simulink model "PassStFtIsPosChk"  (R2024b)
settings: Solver=FixedStepDiscrete  StartTime=0.0  StopTime=10.0  FixedStep=0.01  RelTol=1e-3
model workspace (MAT data in the model file):
  KeSMSuFirstRwStBackPosDelta_Val = Simulink.Parameter
  KeSMSuFirstRwStBackPosDelta_Val.Value = 150
  KeSMSuFirstRwStBackPosDelta_Val.Complexity = 'real'
  KeSMSuFirstRwStBackPosDelta_Val.Dimensions = [1 1]
  KeSMSuFirstRwStBackPosDelta_Val.DataType = 'uint16'
  KeSMSuFirstRwStBackPosTolr_Val = Simulink.Parameter
  KeSMSuFirstRwStBackPosTolr_Val.Value = 150
  KeSMSuFirstRwStBackPosTolr_Val.Complexity = 'real'
  KeSMSuFirstRwStBackPosTolr_Val.Dimensions = [1 1]
  KeSMSuFirstRwStBackPosTolr_Val.DataType = 'uint16'
  KeSMSwAcsMd1PassStCshnRrUpwdDnwdPosMax_Val = Simulink.Parameter
  KeSMSwAcsMd1PassStCshnRrUpwdDnwdPosMax_Val.Value = 0
  KeSMSwAcsMd1PassStCshnRrUpwdDnwdPosMax_Val.Complexity = 'real'
  KeSMSwAcsMd1PassStCshnRrUpwdDnwdPosMax_Val.Dimensions = [1 1]
  KeSMSwAcsMd1PassStCshnRrUpwdDnwdPosMax_Val.DataType = 'uint16'
  KeSMSwAcsMd1PassStCshnRrUpwdDnwdPosMin_Val = Simulink.Parameter
  KeSMSwAcsMd1PassStCshnRrUpwdDnwdPosMin_Val.Value = 0
  KeSMSwAcsMd1PassStCshnRrUpwdDnwdPosMin_Val.Complexity = 'real'
  KeSMSwAcsMd1PassStCshnRrUpwdDnwdPosMin_Val.Dimensions = [1 1]
  KeSMSwAcsMd1PassStCshnRrUpwdDnwdPosMin_Val.DataType = 'uint16'
  KeSMSwAcsMd1PassStCshnRrUpwdDnwdPos_Val = Simulink.Parameter
  KeSMSwAcsMd1PassStCshnRrUpwdDnwdPos_Val.Value = 0
  KeSMSwAcsMd1PassStCshnRrUpwdDnwdPos_Val.Complexity = 'real'
  KeSMSwAcsMd1PassStCshnRrUpwdDnwdPos_Val.Dimensions = [1 1]
  KeSMSwAcsMd1PassStCshnRrUpwdDnwdPos_Val.DataType = 'uint16'
  KeSMSwAcsMd56PassStCshnRrUpwdDnwdPosMax_Val = Simulink.Parameter
  KeSMSwAcsMd56PassStCshnRrUpwdDnwdPosMax_Val.Value = 0
  KeSMSwAcsMd56PassStCshnRrUpwdDnwdPosMax_Val.Complexity = 'real'
  KeSMSwAcsMd56PassStCshnRrUpwdDnwdPosMax_Val.Dimensions = [1 1]
  KeSMSwAcsMd56PassStCshnRrUpwdDnwdPosMax_Val.DataType = 'uint16'
  KeSMSwAcsMd56PassStCshnRrUpwdDnwdPosMin_Val = Simulink.Parameter
  KeSMSwAcsMd56PassStCshnRrUpwdDnwdPosMin_Val.Value = 0
  KeSMSwAcsMd56PassStCshnRrUpwdDnwdPosMin_Val.Complexity = 'real'
  KeSMSwAcsMd56PassStCshnRrUpwdDnwdPosMin_Val.Dimensions = [1 1]
  KeSMSwAcsMd56PassStCshnRrUpwdDnwdPosMin_Val.DataType = 'uint16'
  KeSMSwAcsMd56PassStCshnRrUpwdDnwdPos_Val = Simulink.Parameter
  KeSMSwAcsMd56PassStCshnRrUpwdDnwdPos_Val.Value = 0
  KeSMSwAcsMd56PassStCshnRrUpwdDnwdPos_Val.Complexity = 'real'
  KeSMSwAcsMd56PassStCshnRrUpwdDnwdPos_Val.Dimensions = [1 1]
  KeSMSwAcsMd56PassStCshnRrUpwdDnwdPos_Val.DataType = 'uint16'
undefined symbols (not defined in the file or in its folder): KeSMSuFirstRwStFootrestPosDelta_Val, KeSMSuFirstRwStFootrestPosTolr_Val
libraries: simulink x5, StIsPosChkLib x4
settings Model: ParameterArgumentNames=KeSMSuFirstRwStBackPosDelta_Val,KeSMSuFirstRwStBackPosTolr_Val,KeSMSwAcsMd1PassStCshnRrUpwdDnwdPosMax_Val,KeSMSwAcsMd1PassStCshnRrUpwdDnwdPosMin_Val,KeSMSwAcsMd1PassStCshnRrUpwdDnwdPos_Val,KeSMSwAcsMd56PassStCshnRrUpwdDnwdPosMax_Val,KeSMSwAcsMd56PassStCshnRrUpwdDnwdPosMin_Val,KeSMSwAcsMd56PassStCshnRrUpwdDnwdPos_Val  Creator=sn2xws  LastModifiedBy=sn55gm
settings SolverCC: AlgebraicLoopSolver=TrustRegion
settings DataIOCC: SaveFormat=StructureWithTime  ReturnWorkspaceOutputs=off
settings OptimizationCC: DefaultParameterBehavior=Inlined  EnhancedBackFolding=on  PassReuseOutputArgsAs=Individual arguments  ZeroExternalMemoryAtStartup=off  ZeroInternalMemoryAtStartup=off  OptimizeBlockOrder=speed  DifferentSizesBufferReuse=on  OptimizationCustomize=off  EfficientTunableParamExpr=on
settings DebuggingCC: ParameterTunabilityLossMsg=error  UnconnectedInputMsg=warning  UnconnectedOutputMsg=warning  UnconnectedLineMsg=warning  ArithmeticOperatorsInVariantConditions=warning
settings ModelReferenceCC: EnableRefExpFcnMdlSchedulingChecks=on  ModelReferenceNumInstancesAllowed=Single
settings SFSimCC: MATLABDynamicMemAlloc=off  CustomCodeUndefinedFunction=UseInterfaceOnly
settings RTWCC: Description=AUTOSAR  SystemTargetFile=autosar.tlc  GenCodeOnly=on  TemplateMakefile=ert_default_tmf  GenerateReport=on  IncludeHyperlinkInReport=on  LaunchReport=on  DataTypeReplacement=CDataTypesFixedWidth  GenerateTraceInfo=on  GenerateTraceReport=on  GenerateTraceReportSl=on  GenerateTraceReportSf=on  GenerateTraceReportEml=on  GenerateCodeMetricsReport=on  GPUComputeCapability=3.5
settings CodeAppCC: ForceParamTrailComments=on  IgnoreCustomStorageClasses=off  OperatorAnnotations=on  SimulinkDataObjDesc=on  SFDataObjDesc=on  InsertBlockDesc=on
settings STFCustomTargetCC: TargetLangStandard=C99 (ISO)  MultiwordLength=256  ParMdlRefBuildCompliant=on  CompOptLevelCompliant=on  IncludeMdlTerminateFcn=off  CombineOutputUpdateFcns=on  SuppressErrorStatus=on  ERTCustomFileBanners=on  SupportNonFinite=off  SupportComplex=off  SupportContinuousTime=off  SupportNonInlinedSFcns=off  RemoveResetFunc=on  MATLABClassNameForMDSCustomization=Simulink.SoftwareTarget.ERTCustomization  AutosarCompliant=on  UseToolchainInfoCompliant=on  LookupTableObjectStructAxisOrder=2,1,3,4,...  LUTObjectStructOrderEvenSpacing=Size,Table,Breakpoints  SystemTargetFile=autosar.tlc
settings ERTTargetCC: TargetLangStandard=C99 (ISO)  ConcurrentExecutionCompliant=off  IncludeMdlTerminateFcn=off  SuppressErrorStatus=on  SupportNonFinite=off  SupportComplex=off  ModelStepFunctionPrototypeControlCompliant=off  CPPClassGenCompliant=off  AutosarCompliant=on  LookupTableObjectStructAxisOrder=2,1,3,4,...  LUTObjectStructOrderEvenSpacing=Size,Table,Breakpoints  ERTCustomFileTemplate=example_file_process.tlc  ERTFilePackagingFormat=Compact  BooleanTrueId=TRUE  BooleanFalseId=FALSE  DynamicArrayContainerType=coder::array

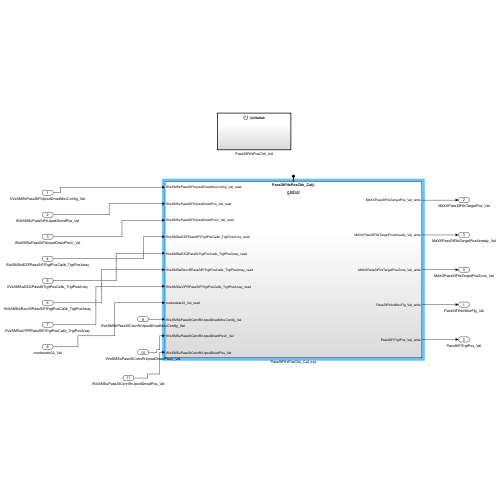
[thumbnail: Simulink's stored preview of the top-level diagram]
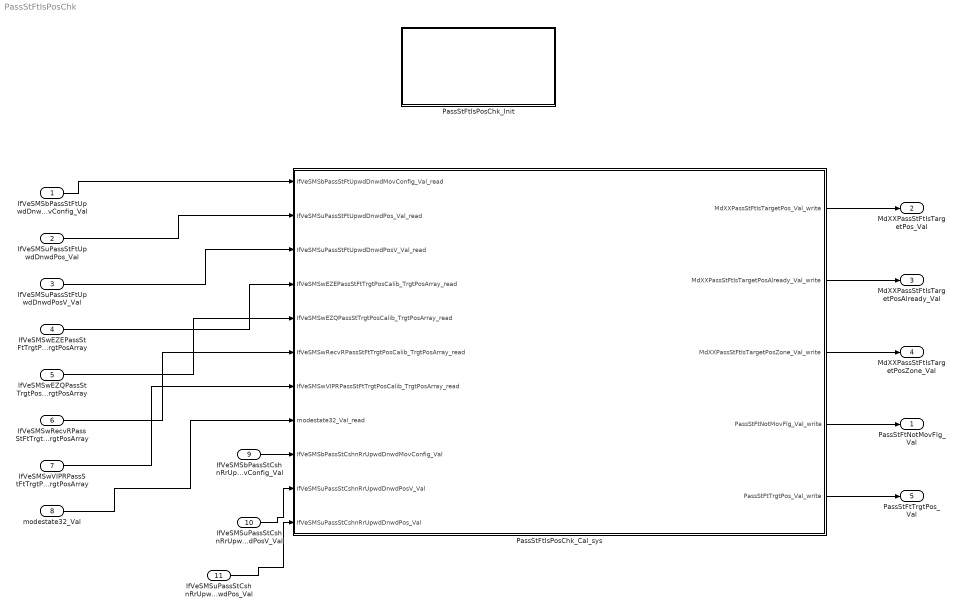
== system PassStFtIsPosChk ==
  IfVeSMSbPassStFtUpwdDnwdMovConfig_Val : Inport  OutDataTypeStr=boolean  PortDimensions=1
  IfVeSMSuPassStFtUpwdDnwdPos_Val : Inport  Port=2  OutDataTypeStr=uint16  PortDimensions=1
  IfVeSMSuPassStFtUpwdDnwdPosV_Val : Inport  Port=3  OutDataTypeStr=boolean  PortDimensions=1
  IfVeSMSwEZEPassStFtTrgtPosCalib_TrgtPosArray : Inport  Description=|  Port=4  OutDataTypeStr=uint16  PortDimensions=3
      | 0:Pos
      | 1:Max
      | 2:Min
  IfVeSMSwEZQPassStTrgtPosCalib_TrgtPosArray : Inport  Description=|  Port=5  OutDataTypeStr=uint16  PortDimensions=3
      | 0:Pos
      | 1:Max
      | 2:Min
  IfVeSMSwRecvRPassStFtTrgtPosCalib_TrgtPosArray : Inport  Description=|  Port=6  OutDataTypeStr=uint16  PortDimensions=3
      | 0:Pos
      | 1:Max
      | 2:Min
  IfVeSMSwVIPRPassStFtTrgtPosCalib_TrgtPosArray : Inport  Description=|  Port=7  OutDataTypeStr=uint16  PortDimensions=3
      | 0:Pos
      | 1:Max
      | 2:Min
  modestate32_Val : Inport  Port=8  OutDataTypeStr=uint32  PortDimensions=1
  IfVeSMSbPassStCshnRrUpwdDnwdMovConfig_Val : Inport  Port=9  OutDataTypeStr=boolean  PortDimensions=1
  IfVeSMSuPassStCshnRrUpwdDnwdPosV_Val : Inport  Port=10  OutDataTypeStr=boolean  PortDimensions=1
  IfVeSMSuPassStCshnRrUpwdDnwdPos_Val : Inport  Port=11  OutDataTypeStr=uint16  PortDimensions=1
  PassStFtIsPosChk_Cal_sys : Subsystem
  PassStFtIsPosChk_Init : Subsystem
  PassStFtNotMovFlg_Val : Outport  OutDataTypeStr=boolean  PortDimensions=1  VectorParamsAs1DForOutWhenUnconnected=off
  MdXXPassStFtIsTargetPos_Val : Outport  Port=2  OutDataTypeStr=uint32  PortDimensions=1  VectorParamsAs1DForOutWhenUnconnected=off
  MdXXPassStFtIsTargetPosAlready_Val : Outport  Port=3  OutDataTypeStr=uint32  PortDimensions=1  VectorParamsAs1DForOutWhenUnconnected=off
  MdXXPassStFtIsTargetPosZone_Val : Outport  Port=4  OutDataTypeStr=uint32  PortDimensions=1  VectorParamsAs1DForOutWhenUnconnected=off
  PassStFtTrgtPos_Val : Outport  Port=5  OutDataTypeStr=uint16  PortDimensions=1  VectorParamsAs1DForOutWhenUnconnected=off
  wires:
  PassStFtIsPosChk_Cal_sys/3(MdXXPassStFtIsTargetPosZone_Val_write) -> MdXXPassStFtIsTargetPosZone_Val/1
  PassStFtIsPosChk_Cal_sys/5(PassStFtTrgtPos_Val_write) -> PassStFtTrgtPos_Val/1
  IfVeSMSuPassStFtUpwdDnwdPosV_Val/1 -> PassStFtIsPosChk_Cal_sys/3(IfVeSMSuPassStFtUpwdDnwdPosV_Val_read)
  IfVeSMSuPassStFtUpwdDnwdPos_Val/1 -> PassStFtIsPosChk_Cal_sys/2(IfVeSMSuPassStFtUpwdDnwdPos_Val_read)
  IfVeSMSwEZEPassStFtTrgtPosCalib_TrgtPosArray/1 -> PassStFtIsPosChk_Cal_sys/4(IfVeSMSwEZEPassStFtTrgtPosCalib_TrgtPosArray_read)
  IfVeSMSbPassStFtUpwdDnwdMovConfig_Val/1 -> PassStFtIsPosChk_Cal_sys/1(IfVeSMSbPassStFtUpwdDnwdMovConfig_Val_read)
  IfVeSMSwEZQPassStTrgtPosCalib_TrgtPosArray/1 -> PassStFtIsPosChk_Cal_sys/5(IfVeSMSwEZQPassStTrgtPosCalib_TrgtPosArray_read)
  IfVeSMSwRecvRPassStFtTrgtPosCalib_TrgtPosArray/1 -> PassStFtIsPosChk_Cal_sys/6(IfVeSMSwRecvRPassStFtTrgtPosCalib_TrgtPosArray_read)
  IfVeSMSwVIPRPassStFtTrgtPosCalib_TrgtPosArray/1 -> PassStFtIsPosChk_Cal_sys/7(IfVeSMSwVIPRPassStFtTrgtPosCalib_TrgtPosArray_read)
  modestate32_Val/1 -> PassStFtIsPosChk_Cal_sys/8(modestate32_Val_read)
  PassStFtIsPosChk_Cal_sys/1(MdXXPassStFtIsTargetPos_Val_write) -> MdXXPassStFtIsTargetPos_Val/1
  PassStFtIsPosChk_Cal_sys/2(MdXXPassStFtIsTargetPosAlready_Val_write) -> MdXXPassStFtIsTargetPosAlready_Val/1
  PassStFtIsPosChk_Cal_sys/4(PassStFtNotMovFlg_Val_write) -> PassStFtNotMovFlg_Val/1
  IfVeSMSbPassStCshnRrUpwdDnwdMovConfig_Val/1 -> PassStFtIsPosChk_Cal_sys/9(IfVeSMSbPassStCshnRrUpwdDnwdMovConfig_Val)
  IfVeSMSuPassStCshnRrUpwdDnwdPosV_Val/1 -> PassStFtIsPosChk_Cal_sys/10(IfVeSMSuPassStCshnRrUpwdDnwdPosV_Val)
  IfVeSMSuPassStCshnRrUpwdDnwdPos_Val/1 -> PassStFtIsPosChk_Cal_sys/11(IfVeSMSuPassStCshnRrUpwdDnwdPos_Val)

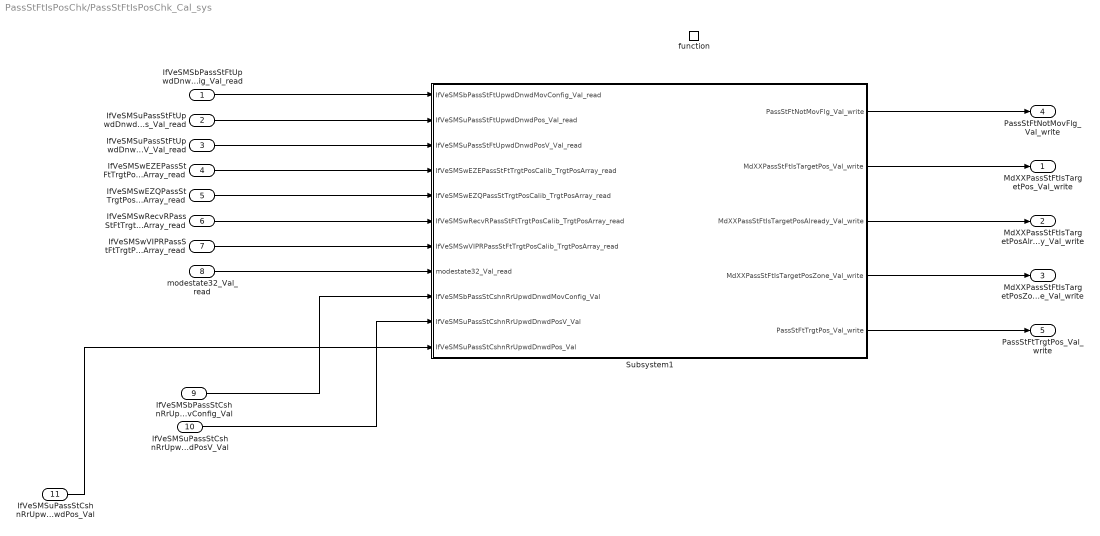
== system PassStFtIsPosChk/PassStFtIsPosChk_Cal_sys ==
  IfVeSMSbPassStFtUpwdDnwdMovConfig_Val_read : Inport
  IfVeSMSuPassStFtUpwdDnwdPos_Val_read : Inport  Port=2
  IfVeSMSuPassStFtUpwdDnwdPosV_Val_read : Inport  Port=3
  IfVeSMSwEZEPassStFtTrgtPosCalib_TrgtPosArray_read : Inport  Port=4
  IfVeSMSwEZQPassStTrgtPosCalib_TrgtPosArray_read : Inport  Port=5
  IfVeSMSwRecvRPassStFtTrgtPosCalib_TrgtPosArray_read : Inport  Port=6
  IfVeSMSwVIPRPassStFtTrgtPosCalib_TrgtPosArray_read : Inport  Port=7
  modestate32_Val_read : Inport  Port=8
  IfVeSMSbPassStCshnRrUpwdDnwdMovConfig_Val : Inport  Port=9
  IfVeSMSuPassStCshnRrUpwdDnwdPosV_Val : Inport  Port=10
  IfVeSMSuPassStCshnRrUpwdDnwdPos_Val : Inport  Port=11
  function : TriggerPort  TriggerType=function-call  IsSimulinkFunction=on  FunctionName=PassStFtIsPosChk_Cal  VariantControl=(inherit)
  Subsystem1 : Subsystem
  MdXXPassStFtIsTargetPos_Val_write : Outport  VectorParamsAs1DForOutWhenUnconnected=off
      settings: EnsureOutportIsVirtual=on
  MdXXPassStFtIsTargetPosAlready_Val_write : Outport  Port=2  VectorParamsAs1DForOutWhenUnconnected=off
      settings: EnsureOutportIsVirtual=on
  MdXXPassStFtIsTargetPosZone_Val_write : Outport  Port=3  VectorParamsAs1DForOutWhenUnconnected=off
      settings: EnsureOutportIsVirtual=on
  PassStFtNotMovFlg_Val_write : Outport  Port=4  VectorParamsAs1DForOutWhenUnconnected=off
      settings: EnsureOutportIsVirtual=on
  PassStFtTrgtPos_Val_write : Outport  Port=5  VectorParamsAs1DForOutWhenUnconnected=off
      settings: EnsureOutportIsVirtual=on
  wires:
  IfVeSMSwEZQPassStTrgtPosCalib_TrgtPosArray_read/1 -> Subsystem1/5(IfVeSMSwEZQPassStTrgtPosCalib_TrgtPosArray_read)
  IfVeSMSwRecvRPassStFtTrgtPosCalib_TrgtPosArray_read/1 -> Subsystem1/6(IfVeSMSwRecvRPassStFtTrgtPosCalib_TrgtPosArray_read)
  IfVeSMSuPassStFtUpwdDnwdPosV_Val_read/1 -> Subsystem1/3(IfVeSMSuPassStFtUpwdDnwdPosV_Val_read)
  IfVeSMSwEZEPassStFtTrgtPosCalib_TrgtPosArray_read/1 -> Subsystem1/4(IfVeSMSwEZEPassStFtTrgtPosCalib_TrgtPosArray_read)
  IfVeSMSwVIPRPassStFtTrgtPosCalib_TrgtPosArray_read/1 -> Subsystem1/7(IfVeSMSwVIPRPassStFtTrgtPosCalib_TrgtPosArray_read)
  IfVeSMSuPassStFtUpwdDnwdPos_Val_read/1 -> Subsystem1/2(IfVeSMSuPassStFtUpwdDnwdPos_Val_read)
  modestate32_Val_read/1 -> Subsystem1/8(modestate32_Val_read)
  IfVeSMSbPassStFtUpwdDnwdMovConfig_Val_read/1 -> Subsystem1/1(IfVeSMSbPassStFtUpwdDnwdMovConfig_Val_read)
  Subsystem1/1(PassStFtNotMovFlg_Val_write) -> PassStFtNotMovFlg_Val_write/1
  Subsystem1/2(MdXXPassStFtIsTargetPos_Val_write) -> MdXXPassStFtIsTargetPos_Val_write/1
  Subsystem1/3(MdXXPassStFtIsTargetPosAlready_Val_write) -> MdXXPassStFtIsTargetPosAlready_Val_write/1
  Subsystem1/4(MdXXPassStFtIsTargetPosZone_Val_write) -> MdXXPassStFtIsTargetPosZone_Val_write/1
  Subsystem1/5(PassStFtTrgtPos_Val_write) -> PassStFtTrgtPos_Val_write/1
  IfVeSMSbPassStCshnRrUpwdDnwdMovConfig_Val/1 -> Subsystem1/9(IfVeSMSbPassStCshnRrUpwdDnwdMovConfig_Val)
  IfVeSMSuPassStCshnRrUpwdDnwdPosV_Val/1 -> Subsystem1/10(IfVeSMSuPassStCshnRrUpwdDnwdPosV_Val)
  IfVeSMSuPassStCshnRrUpwdDnwdPos_Val/1 -> Subsystem1/11(IfVeSMSuPassStCshnRrUpwdDnwdPos_Val)

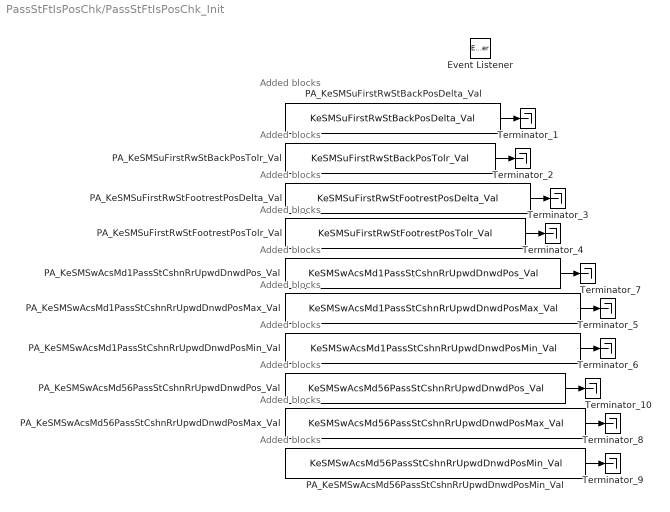
== system PassStFtIsPosChk/PassStFtIsPosChk_Init ==
  note: Added blocks
  note: Added blocks
  note: Added blocks
  note: Added blocks
  note: Added blocks
  note: Added blocks
  note: Added blocks
  note: Added blocks
  note: Added blocks
  note: Added blocks
  Event Listener : EventListener  EventName=reset
  PA_KeSMSuFirstRwStBackPosDelta_Val : Constant  Value=KeSMSuFirstRwStBackPosDelta_Val
  PA_KeSMSuFirstRwStBackPosTolr_Val : Constant  Value=KeSMSuFirstRwStBackPosTolr_Val
  PA_KeSMSuFirstRwStFootrestPosDelta_Val : Constant  Value=KeSMSuFirstRwStFootrestPosDelta_Val
  PA_KeSMSuFirstRwStFootrestPosTolr_Val : Constant  Value=KeSMSuFirstRwStFootrestPosTolr_Val
  PA_KeSMSwAcsMd1PassStCshnRrUpwdDnwdPosMax_Val : Constant  Value=KeSMSwAcsMd1PassStCshnRrUpwdDnwdPosMax_Val
  PA_KeSMSwAcsMd1PassStCshnRrUpwdDnwdPosMin_Val : Constant  Value=KeSMSwAcsMd1PassStCshnRrUpwdDnwdPosMin_Val
  PA_KeSMSwAcsMd1PassStCshnRrUpwdDnwdPos_Val : Constant  Value=KeSMSwAcsMd1PassStCshnRrUpwdDnwdPos_Val
  PA_KeSMSwAcsMd56PassStCshnRrUpwdDnwdPosMax_Val : Constant  Value=KeSMSwAcsMd56PassStCshnRrUpwdDnwdPosMax_Val
  PA_KeSMSwAcsMd56PassStCshnRrUpwdDnwdPosMin_Val : Constant  Value=KeSMSwAcsMd56PassStCshnRrUpwdDnwdPosMin_Val
  PA_KeSMSwAcsMd56PassStCshnRrUpwdDnwdPos_Val : Constant  Value=KeSMSwAcsMd56PassStCshnRrUpwdDnwdPos_Val
  Terminator_{1..10} (10 alike) : Terminator
  wires:
  PA_KeSMSuFirstRwStBackPosDelta_Val/1 -> Terminator_1/1
  PA_KeSMSuFirstRwStBackPosTolr_Val/1 -> Terminator_2/1
  PA_KeSMSuFirstRwStFootrestPosDelta_Val/1 -> Terminator_3/1
  PA_KeSMSuFirstRwStFootrestPosTolr_Val/1 -> Terminator_4/1
  PA_KeSMSwAcsMd1PassStCshnRrUpwdDnwdPosMax_Val/1 -> Terminator_5/1
  PA_KeSMSwAcsMd1PassStCshnRrUpwdDnwdPosMin_Val/1 -> Terminator_6/1
  PA_KeSMSwAcsMd1PassStCshnRrUpwdDnwdPos_Val/1 -> Terminator_7/1
  PA_KeSMSwAcsMd56PassStCshnRrUpwdDnwdPosMax_Val/1 -> Terminator_8/1
  PA_KeSMSwAcsMd56PassStCshnRrUpwdDnwdPosMin_Val/1 -> Terminator_9/1
  PA_KeSMSwAcsMd56PassStCshnRrUpwdDnwdPos_Val/1 -> Terminator_10/1

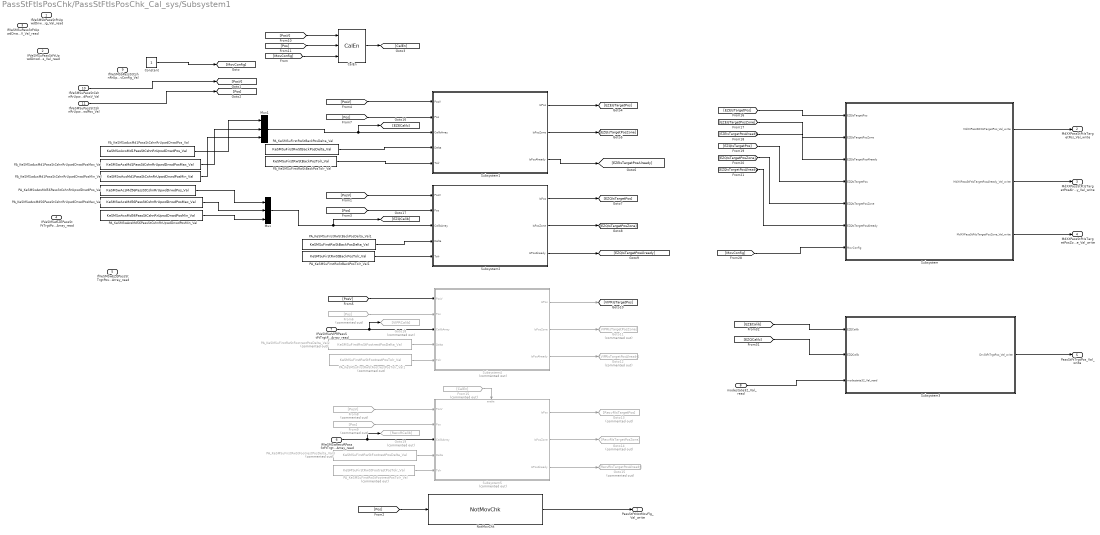
== system PassStFtIsPosChk/PassStFtIsPosChk_Cal_sys/Subsystem1 ==
  IfVeSMSbPassStFtUpwdDnwdMovConfig_Val_read : Inport
  IfVeSMSuPassStFtUpwdDnwdPos_Val_read : Inport  Port=2
  IfVeSMSuPassStFtUpwdDnwdPosV_Val_read : Inport  Port=3
  IfVeSMSwEZEPassStFtTrgtPosCalib_TrgtPosArray_read : Inport  Port=4
  IfVeSMSwEZQPassStTrgtPosCalib_TrgtPosArray_read : Inport  Port=5
  IfVeSMSwRecvRPassStFtTrgtPosCalib_TrgtPosArray_read : Inport  Port=6
  IfVeSMSwVIPRPassStFtTrgtPosCalib_TrgtPosArray_read : Inport  Port=7
  modestate32_Val_read : Inport  Port=8
  IfVeSMSbPassStCshnRrUpwdDnwdMovConfig_Val : Inport  Port=9
  IfVeSMSuPassStCshnRrUpwdDnwdPosV_Val : Inport  Port=10
  IfVeSMSuPassStCshnRrUpwdDnwdPos_Val : Inport  Port=11
  CalEn : StIsPosChkLib/CalEn  SystemSampleTime=-1  VariantActivationTime=update diagram  AllowFlexibleInterface=on  Latency=0  AutoFrameSizeCalculation=off
  Constant : Constant
  From15 : From  Commented=on  GotoTag=CalEn
  From6 : From  Commented=on  GotoTag=Pos
  From8 : From  Commented=on  GotoTag=PosV
  From9 : From  Commented=on  GotoTag=Pos
  Goto11 : Goto  Commented=on  GotoTag=VIPRIsTargetPosZone
  Goto12 : Goto  Commented=on  GotoTag=VIPRIsTargetPosAlready
  Goto13 : Goto  Commented=on  GotoTag=RecvRIsTargetPos
  Goto14 : Goto  Commented=on  GotoTag=RecvRIsTargetPosZone
  Goto15 : Goto  Commented=on  GotoTag=RecvRIsTargetPosAlready
  Goto18 : Goto  Commented=on  GotoTag=VIPRCalib
  Goto19 : Goto  Commented=on  GotoTag=RecvRCalib
  Mux : Mux  Inputs=3
  Mux1 : Mux  Inputs=3
  NotMovChk : StIsPosChkLib/NotMovChk  SystemSampleTime=-1  VariantActivationTime=update diagram  AllowFlexibleInterface=on  Latency=0  AutoFrameSizeCalculation=off
  PA_KeSMSuFirstRwStBackPosDelta_Val : Constant  Value=KeSMSuFirstRwStBackPosDelta_Val
  PA_KeSMSuFirstRwStBackPosDelta_Val1 : Constant  Value=KeSMSuFirstRwStBackPosDelta_Val
  PA_KeSMSuFirstRwStBackPosTolr_Val : Constant  Value=KeSMSuFirstRwStBackPosTolr_Val
  PA_KeSMSuFirstRwStBackPosTolr_Val1 : Constant  Value=KeSMSuFirstRwStBackPosTolr_Val
  PA_KeSMSuFirstRwStFootrestPosDelta_Val2 : Constant  Commented=on  Value=KeSMSuFirstRwStFootrestPosDelta_Val
  PA_KeSMSuFirstRwStFootrestPosDelta_Val3 : Constant  Commented=on  Value=KeSMSuFirstRwStFootrestPosDelta_Val
  PA_KeSMSuFirstRwStFootrestPosTolr_Val : Constant  Commented=on  Value=KeSMSuFirstRwStFootrestPosTolr_Val
  PA_KeSMSuFirstRwStFootrestPosTolr_Val1 : Constant  Commented=on  Value=KeSMSuFirstRwStFootrestPosTolr_Val
  PA_KeSMSwAcsMd1PassStCshnRrUpwdDnwdPosMax_Val : Constant  Value=KeSMSwAcsMd1PassStCshnRrUpwdDnwdPosMax_Val
  PA_KeSMSwAcsMd1PassStCshnRrUpwdDnwdPosMin_Val : Constant  Value=KeSMSwAcsMd1PassStCshnRrUpwdDnwdPosMin_Val
  PA_KeSMSwAcsMd1PassStCshnRrUpwdDnwdPos_Val : Constant  Value=KeSMSwAcsMd1PassStCshnRrUpwdDnwdPos_Val
  PA_KeSMSwAcsMd56PassStCshnRrUpwdDnwdPosMax_Val : Constant  Value=KeSMSwAcsMd56PassStCshnRrUpwdDnwdPosMax_Val
  PA_KeSMSwAcsMd56PassStCshnRrUpwdDnwdPosMin_Val : Constant  Value=KeSMSwAcsMd56PassStCshnRrUpwdDnwdPosMin_Val
  PA_KeSMSwAcsMd56PassStCshnRrUpwdDnwdPos_Val : Constant  Value=KeSMSwAcsMd56PassStCshnRrUpwdDnwdPos_Val
  Subsystem : Subsystem
  Subsystem1 : Subsystem
  Subsystem2 : Subsystem
  Subsystem3 : Subsystem
  Subsystem4 : Subsystem  Commented=on
  Subsystem5 : Subsystem  Commented=on
  PassStFtNotMovFlg_Val_write : Outport  VectorParamsAs1DForOutWhenUnconnected=off
      settings: EnsureOutportIsVirtual=on
  MdXXPassStFtIsTargetPos_Val_write : Outport  Port=2  VectorParamsAs1DForOutWhenUnconnected=off
      settings: EnsureOutportIsVirtual=on
  MdXXPassStFtIsTargetPosAlready_Val_write : Outport  Port=3  VectorParamsAs1DForOutWhenUnconnected=off
      settings: EnsureOutportIsVirtual=on
  MdXXPassStFtIsTargetPosZone_Val_write : Outport  Port=4  VectorParamsAs1DForOutWhenUnconnected=off
      settings: EnsureOutportIsVirtual=on
  PassStFtTrgtPos_Val_write : Outport  Port=5  VectorParamsAs1DForOutWhenUnconnected=off
      settings: EnsureOutportIsVirtual=on
  wires:
  Subsystem2/3(IsPosAlready) -> [EZQIsTargetPosAlready]
  PA_KeSMSuFirstRwStFootrestPosTolr_Val1/1 -> Subsystem4/5(Tolr)
  PA_KeSMSuFirstRwStFootrestPosTolr_Val/1 -> Subsystem5/5(Tolr)
  Subsystem3/1(DrvStFtTrgtPos_Val_write) -> PassStFtTrgtPos_Val_write/1
  PA_KeSMSuFirstRwStFootrestPosDelta_Val3/1 -> Subsystem5/4(Delta)
  [EZEIsTargetPos] -> Subsystem/1(EZEIsTargetPos)
  [PosV] -> Subsystem4/1(PosV)
  [EZQCalib] -> Subsystem3/2(EZQCalib)
  modestate32_Val_read/1 -> Subsystem3/3(modestate32_Val_read)
  [MovConfig] -> Subsystem/7(MovConfig)
  PA_KeSMSuFirstRwStBackPosTolr_Val1/1 -> Subsystem2/5(Tolr)
  [EZQIsTargetPosAlready] -> Subsystem/6(EZQIsTargetPosAlready)
  [Pos] -> NotMovChk/1
  From9/1 -> Subsystem5/2(Pos)
  Subsystem2/1(IsPos) -> [EZQIsTargetPos]
  IfVeSMSwVIPRPassStFtTrgtPosCalib_TrgtPosArray_read/1 -> Subsystem4/3(CalibArray), Goto18/1
  Subsystem5/3(IsPosAlready) -> Goto15/1
  [EZQIsTargetPos] -> Subsystem/4(EZQIsTargetPos)
  Subsystem4/3(IsPosAlready) -> Goto12/1
  From8/1 -> Subsystem5/1(PosV)
  Subsystem4/1(IsPos) -> [VIPRIsTargetPos]
  Subsystem1/1(IsPos) -> [EZEIsTargetPos]
  Subsystem1/2(IsPosZone) -> [EZEIsTargetPosZone]
  From15/1 -> Subsystem5/Enable
  [PosV] -> CalEn/1
  NotMovChk/1 -> PassStFtNotMovFlg_Val_write/1
  PA_KeSMSuFirstRwStBackPosTolr_Val/1 -> Subsystem1/5(Tolr)
  From6/1 -> Subsystem4/2(Pos)
  [Pos] -> CalEn/2
  [EZECalib] -> Subsystem3/1(EZECalib)
  [EZQIsTargetPosZone] -> Subsystem/5(EZQIsTargetPosZone)
  Subsystem1/3(IsPosAlready) -> [EZEIsTargetPosAlready]
  [Pos] -> Subsystem2/2(Pos)
  [Pos] -> Subsystem1/2(Pos)
  PA_KeSMSuFirstRwStBackPosDelta_Val1/1 -> Subsystem2/4(Delta)
  [MovConfig] -> CalEn/3
  [PosV] -> Subsystem2/1(PosV)
  [PosV] -> Subsystem1/1(PosV)
  IfVeSMSwRecvRPassStFtTrgtPosCalib_TrgtPosArray_read/1 -> Subsystem5/3(CalibArray), Goto19/1
  CalEn/1 -> [CalEn]
  PA_KeSMSuFirstRwStFootrestPosDelta_Val2/1 -> Subsystem4/4(Delta)
  Subsystem4/2(IsPosZone) -> Goto11/1
  [EZEIsTargetPosZone] -> Subsystem/2(EZEIsTargetPosZone)
  Subsystem5/1(IsPos) -> Goto13/1
  Subsystem/2(MdXXPassStFtIsTargetPosAlready_Val_write) -> MdXXPassStFtIsTargetPosAlready_Val_write/1
  Subsystem/3(MdXXPassStFtIsTargetPosZone_Val_write) -> MdXXPassStFtIsTargetPosZone_Val_write/1
  Subsystem5/2(IsPosZone) -> Goto14/1
  Subsystem/1(MdXXPassStFtIsTargetPos_Val_write) -> MdXXPassStFtIsTargetPos_Val_write/1
  Subsystem2/2(IsPosZone) -> [EZQIsTargetPosZone]
  [EZEIsTargetPosAlready] -> Subsystem/3(EZEIsTargetPosAlready)
  PA_KeSMSuFirstRwStBackPosDelta_Val/1 -> Subsystem1/4(Delta)
  PA_KeSMSwAcsMd1PassStCshnRrUpwdDnwdPosMax_Val/1 -> Mux1/2
  PA_KeSMSwAcsMd1PassStCshnRrUpwdDnwdPosMin_Val/1 -> Mux1/3
  PA_KeSMSwAcsMd1PassStCshnRrUpwdDnwdPos_Val/1 -> Mux1/1
  PA_KeSMSwAcsMd56PassStCshnRrUpwdDnwdPos_Val/1 -> Mux/1
  IfVeSMSuPassStCshnRrUpwdDnwdPosV_Val/1 -> [PosV]
  IfVeSMSuPassStCshnRrUpwdDnwdPos_Val/1 -> [Pos]
  PA_KeSMSwAcsMd56PassStCshnRrUpwdDnwdPosMax_Val/1 -> Mux/2
  PA_KeSMSwAcsMd56PassStCshnRrUpwdDnwdPosMin_Val/1 -> Mux/3
  Mux/1 -> [EZQCalib], Subsystem2/3(CalibArray)
  Mux1/1 -> [EZECalib], Subsystem1/3(CalibArray)
  Constant/1 -> [MovConfig]

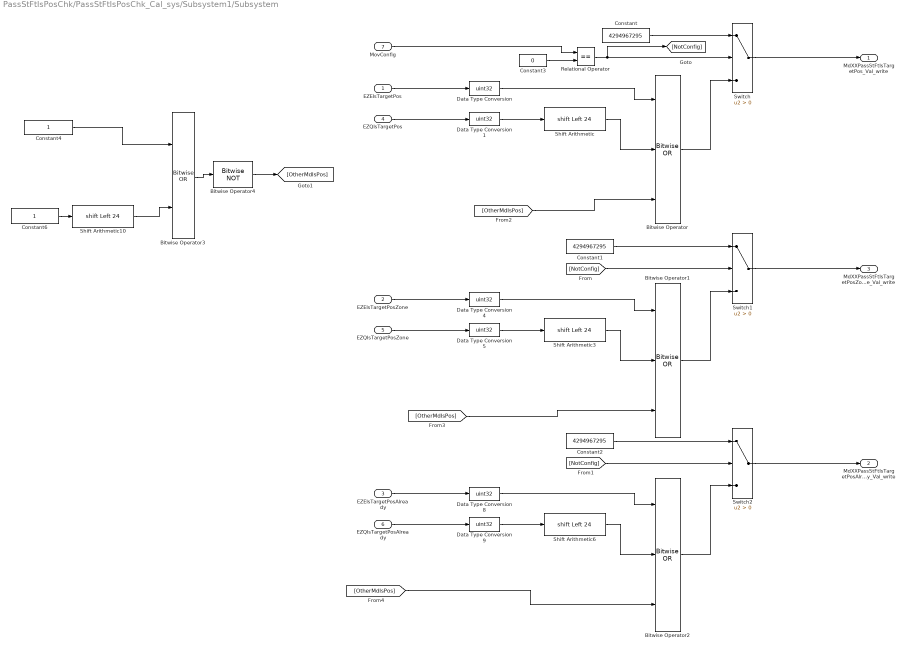
== system PassStFtIsPosChk/PassStFtIsPosChk_Cal_sys/Subsystem1/Subsystem ==
  EZEIsTargetPos : Inport
  EZEIsTargetPosZone : Inport  Port=2
  EZEIsTargetPosAlready : Inport  Port=3
  EZQIsTargetPos : Inport  Port=4
  EZQIsTargetPosZone : Inport  Port=5
  EZQIsTargetPosAlready : Inport  Port=6
  MovConfig : Inport  Port=7
  Bitwise Operator : simulink/Logic and Bit Operations/Bitwise Operator  logicop=OR  UseBitMask=off  NumInputPorts=3  BitMask=bin2dec('11011001')  BitMaskRealWorld=Stored Integer
  Bitwise Operator1 : simulink/Logic and Bit Operations/Bitwise Operator  logicop=OR  UseBitMask=off  NumInputPorts=3  BitMask=bin2dec('11011001')  BitMaskRealWorld=Stored Integer
  Bitwise Operator2 : simulink/Logic and Bit Operations/Bitwise Operator  logicop=OR  UseBitMask=off  NumInputPorts=3  BitMask=bin2dec('11011001')  BitMaskRealWorld=Stored Integer
  Bitwise Operator3 : simulink/Logic and Bit Operations/Bitwise Operator  logicop=OR  UseBitMask=off  NumInputPorts=2  BitMask=bin2dec('11011001')  BitMaskRealWorld=Stored Integer
  Bitwise Operator4 : simulink/Logic and Bit Operations/Bitwise Operator  logicop=NOT  UseBitMask=off  BitMask=bin2dec('11011001')  BitMaskRealWorld=Stored Integer
  Constant : Constant  Value=4294967295  OutDataTypeStr=uint32
  Constant1 : Constant  Value=4294967295  OutDataTypeStr=uint32
  Constant2 : Constant  Value=4294967295  OutDataTypeStr=uint32
  Constant3 : Constant  Value=0  OutDataTypeStr=uint8
  Constant4 : Constant  OutDataTypeStr=uint32
  Constant6 : Constant  OutDataTypeStr=uint32
  Data Type Conversion{,1,4..5,8..9} (6 alike) : DataTypeConversion  OutDataTypeStr=uint32  SaturateOnIntegerOverflow=off  RndMeth=Floor
  Relational Operator : RelationalOperator  Operator===  OutDataTypeStr=boolean  RndMeth=Simplest  InputSameDT=off
  Shift Arithmetic{,3,6,10} (4 alike) : ArithShift  BitShiftNumber=24  BitShiftDirection=Left
  Switch : Switch  Criteria=u2 > Threshold  SaturateOnIntegerOverflow=off  InputSameDT=off
  Switch1 : Switch  Criteria=u2 > Threshold  SaturateOnIntegerOverflow=off  InputSameDT=off
  Switch2 : Switch  Criteria=u2 > Threshold  SaturateOnIntegerOverflow=off  InputSameDT=off
  MdXXPassStFtIsTargetPos_Val_write : Outport  VectorParamsAs1DForOutWhenUnconnected=off
      settings: EnsureOutportIsVirtual=on
  MdXXPassStFtIsTargetPosAlready_Val_write : Outport  Port=2  VectorParamsAs1DForOutWhenUnconnected=off
      settings: EnsureOutportIsVirtual=on
  MdXXPassStFtIsTargetPosZone_Val_write : Outport  Port=3  VectorParamsAs1DForOutWhenUnconnected=off
      settings: EnsureOutportIsVirtual=on
  wires:
  Constant3/1 -> Relational Operator/2
  Shift Arithmetic/1 -> Bitwise Operator/2
  MovConfig/1 -> Relational Operator/1
  Bitwise Operator/1 -> Switch/3
  Data Type Conversion1/1 -> Shift Arithmetic/1
  Relational Operator/1 -> [NotConfig], Switch/2
  EZQIsTargetPos/1 -> Data Type Conversion1/1
  Data Type Conversion/1 -> Bitwise Operator/1
  Constant/1 -> Switch/1
  EZEIsTargetPos/1 -> Data Type Conversion/1
  Switch/1 -> MdXXPassStFtIsTargetPos_Val_write/1
  EZEIsTargetPosZone/1 -> Data Type Conversion4/1
  Constant1/1 -> Switch1/1
  Data Type Conversion4/1 -> Bitwise Operator1/1
  EZQIsTargetPosZone/1 -> Data Type Conversion5/1
  Data Type Conversion5/1 -> Shift Arithmetic3/1
  Bitwise Operator1/1 -> Switch1/3
  Shift Arithmetic3/1 -> Bitwise Operator1/2
  [NotConfig] -> Switch1/2
  [NotConfig] -> Switch2/2
  Shift Arithmetic6/1 -> Bitwise Operator2/2
  Bitwise Operator2/1 -> Switch2/3
  Data Type Conversion9/1 -> Shift Arithmetic6/1
  EZQIsTargetPosAlready/1 -> Data Type Conversion9/1
  Data Type Conversion8/1 -> Bitwise Operator2/1
  Constant2/1 -> Switch2/1
  EZEIsTargetPosAlready/1 -> Data Type Conversion8/1
  Switch2/1 -> MdXXPassStFtIsTargetPosAlready_Val_write/1
  Switch1/1 -> MdXXPassStFtIsTargetPosZone_Val_write/1
  Constant4/1 -> Bitwise Operator3/1
  Constant6/1 -> Shift Arithmetic10/1
  Shift Arithmetic10/1 -> Bitwise Operator3/2
  Bitwise Operator3/1 -> Bitwise Operator4/1
  Bitwise Operator4/1 -> [OtherMdIsPos]
  [OtherMdIsPos] -> Bitwise Operator/3
  [OtherMdIsPos] -> Bitwise Operator1/3
  [OtherMdIsPos] -> Bitwise Operator2/3

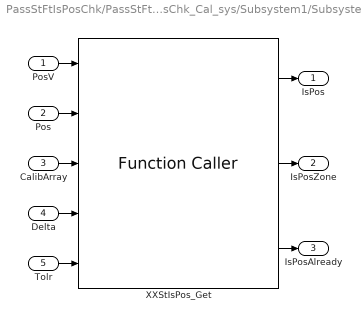
== system PassStFtIsPosChk/PassStFtIsPosChk_Cal_sys/Subsystem1/Subsystem1 ==
  PosV : Inport
  Pos : Inport  Port=2
  CalibArray : Inport  Port=3
  Delta : Inport  Port=4
  Tolr : Inport  Port=5
  XXStIsPos_Get : FunctionCaller  FunctionPrototype=[IsPos,IsPosZone,IsPosAlready] = XXStIsPos_Get(PosV,Pos,CalibArray,Delta,Tolr)  InputArgumentSpecifications=boolean(true), uint16(1), uint16([1;1;1]), uint16(1), uint16(1)  OutputArgumentSpecifications=boolean(true), boolean(true), boolean(true)
  IsPos : Outport  VectorParamsAs1DForOutWhenUnconnected=off
  IsPosZone : Outport  Port=2  VectorParamsAs1DForOutWhenUnconnected=off
  IsPosAlready : Outport  Port=3  VectorParamsAs1DForOutWhenUnconnected=off
  wires:
  PosV/1 -> XXStIsPos_Get/1
  XXStIsPos_Get/3 -> IsPosAlready/1
  Tolr/1 -> XXStIsPos_Get/5
  XXStIsPos_Get/1 -> IsPos/1
  XXStIsPos_Get/2 -> IsPosZone/1
  CalibArray/1 -> XXStIsPos_Get/3
  Delta/1 -> XXStIsPos_Get/4
  Pos/1 -> XXStIsPos_Get/2

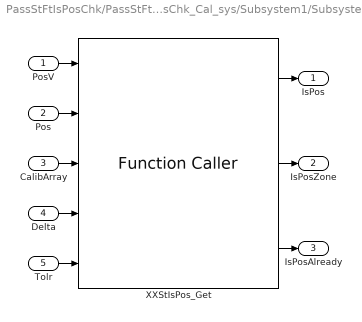
== system PassStFtIsPosChk/PassStFtIsPosChk_Cal_sys/Subsystem1/Subsystem2 ==
  PosV : Inport
  Pos : Inport  Port=2
  CalibArray : Inport  Port=3
  Delta : Inport  Port=4
  Tolr : Inport  Port=5
  XXStIsPos_Get : FunctionCaller  FunctionPrototype=[IsPos,IsPosZone,IsPosAlready] = XXStIsPos_Get(PosV,Pos,CalibArray,Delta,Tolr)  InputArgumentSpecifications=boolean(true), uint16(1), uint16([1;1;1]), uint16(1), uint16(1)  OutputArgumentSpecifications=boolean(true), boolean(true), boolean(true)
  IsPos : Outport  VectorParamsAs1DForOutWhenUnconnected=off
  IsPosZone : Outport  Port=2  VectorParamsAs1DForOutWhenUnconnected=off
  IsPosAlready : Outport  Port=3  VectorParamsAs1DForOutWhenUnconnected=off
  wires:
  Pos/1 -> XXStIsPos_Get/2
  Delta/1 -> XXStIsPos_Get/4
  CalibArray/1 -> XXStIsPos_Get/3
  XXStIsPos_Get/2 -> IsPosZone/1
  XXStIsPos_Get/1 -> IsPos/1
  Tolr/1 -> XXStIsPos_Get/5
  XXStIsPos_Get/3 -> IsPosAlready/1
  PosV/1 -> XXStIsPos_Get/1

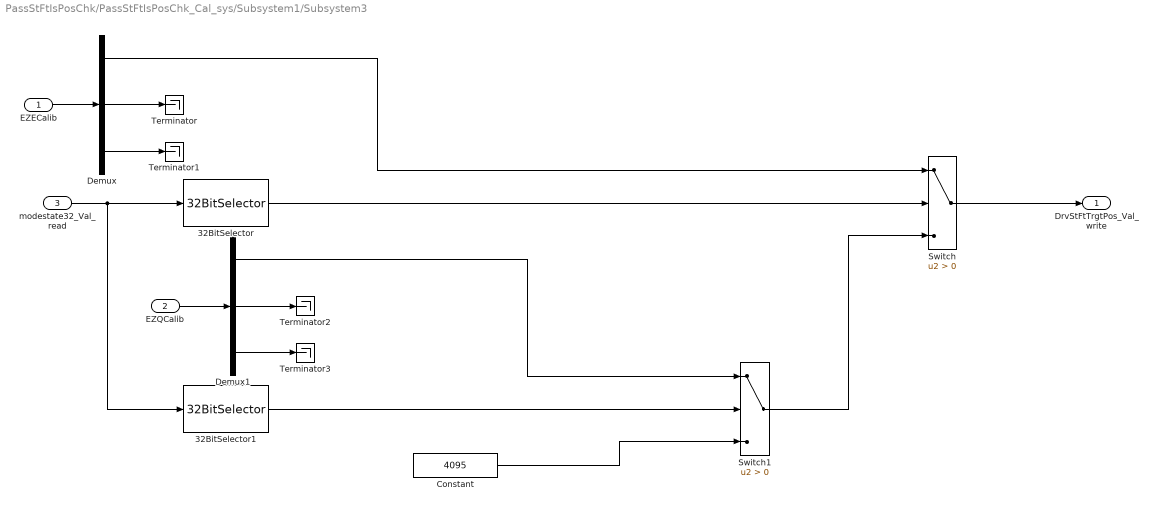
== system PassStFtIsPosChk/PassStFtIsPosChk_Cal_sys/Subsystem1/Subsystem3 ==
  EZECalib : Inport
  EZQCalib : Inport  Port=2
  modestate32_Val_read : Inport  Port=3
  32BitSelector : StIsPosChkLib/32BitSelector  BitNum=0
  32BitSelector1 : StIsPosChkLib/32BitSelector  BitNum=24
  Constant : Constant  Value=4095  OutDataTypeStr=uint16
  Demux : Demux  Outputs=3
  Demux1 : Demux  Outputs=3
  Switch : Switch  Criteria=u2 > Threshold  SaturateOnIntegerOverflow=off  InputSameDT=off
  Switch1 : Switch  Criteria=u2 > Threshold  SaturateOnIntegerOverflow=off  InputSameDT=off
  Terminator{,1..3} (4 alike) : Terminator
  DrvStFtTrgtPos_Val_write : Outport  VectorParamsAs1DForOutWhenUnconnected=off
      settings: EnsureOutportIsVirtual=on
  wires:
  EZECalib/1 -> Demux/1
  Demux/3 -> Terminator1/1
  Demux/2 -> Terminator/1
  Demux1/2 -> Terminator2/1
  Demux1/3 -> Terminator3/1
  EZQCalib/1 -> Demux1/1
  modestate32_Val_read/1 -> 32BitSelector1/1, 32BitSelector/1
  32BitSelector/1 -> Switch/2
  Demux/1 -> Switch/1
  Switch/1 -> DrvStFtTrgtPos_Val_write/1
  Switch1/1 -> Switch/3
  32BitSelector1/1 -> Switch1/2
  Demux1/1 -> Switch1/1
  Constant/1 -> Switch1/3

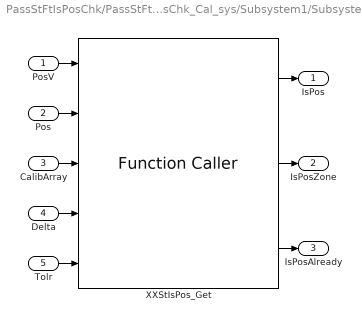
== system PassStFtIsPosChk/PassStFtIsPosChk_Cal_sys/Subsystem1/Subsystem4 ==
  PosV : Inport
  Pos : Inport  Port=2
  CalibArray : Inport  Port=3
  Delta : Inport  Port=4
  Tolr : Inport  Port=5
  XXStIsPos_Get : FunctionCaller  FunctionPrototype=[IsPos,IsPosZone,IsPosAlready] = XXStIsPos_Get(PosV,Pos,CalibArray,Delta,Tolr)  InputArgumentSpecifications=boolean(true), uint16(1), uint16([1;1;1]), uint16(1), uint16(1)  OutputArgumentSpecifications=boolean(true), boolean(true), boolean(true)
  IsPos : Outport  VectorParamsAs1DForOutWhenUnconnected=off
  IsPosZone : Outport  Port=2  VectorParamsAs1DForOutWhenUnconnected=off
  IsPosAlready : Outport  Port=3  VectorParamsAs1DForOutWhenUnconnected=off
  wires:
  PosV/1 -> XXStIsPos_Get/1
  XXStIsPos_Get/3 -> IsPosAlready/1
  Tolr/1 -> XXStIsPos_Get/5
  XXStIsPos_Get/1 -> IsPos/1
  XXStIsPos_Get/2 -> IsPosZone/1
  CalibArray/1 -> XXStIsPos_Get/3
  Delta/1 -> XXStIsPos_Get/4
  Pos/1 -> XXStIsPos_Get/2

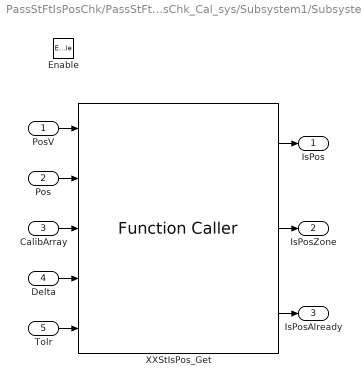
== system PassStFtIsPosChk/PassStFtIsPosChk_Cal_sys/Subsystem1/Subsystem5 ==
  PosV : Inport
  Pos : Inport  Port=2
  CalibArray : Inport  Port=3
  Delta : Inport  Port=4
  Tolr : Inport  Port=5
  Enable : EnablePort
  XXStIsPos_Get : FunctionCaller  FunctionPrototype=[IsPos,IsPosZone,IsPosAlready] = XXStIsPos_Get(PosV,Pos,CalibArray,Delta,Tolr)  InputArgumentSpecifications=boolean(true), uint16(1), uint16([1;1;1]), uint16(1), uint16(1)  OutputArgumentSpecifications=boolean(true), boolean(true), boolean(true)
  IsPos : Outport  VectorParamsAs1DForOutWhenUnconnected=off
  IsPosZone : Outport  Port=2  VectorParamsAs1DForOutWhenUnconnected=off
  IsPosAlready : Outport  Port=3  VectorParamsAs1DForOutWhenUnconnected=off
  wires:
  Pos/1 -> XXStIsPos_Get/2
  Delta/1 -> XXStIsPos_Get/4
  CalibArray/1 -> XXStIsPos_Get/3
  XXStIsPos_Get/2 -> IsPosZone/1
  XXStIsPos_Get/1 -> IsPos/1
  Tolr/1 -> XXStIsPos_Get/5
  XXStIsPos_Get/3 -> IsPosAlready/1
  PosV/1 -> XXStIsPos_Get/1
